simulink model "rlMADDPG4PFC2"  (R2024b)
settings: Solver=FixedStepAuto  StartTime=0.0  StopTime=Tf  FixedStep=0.001  RelTol=1e-3
StartFcn:
  | %scopes= find_system(bdroot,'BlockType','Scope');
  | %for i = 1:length(scopes)
  | %set_param(scopes{i},'Open','on');
  | %end
values from neighbouring files (symbols this model uses):
  amax_ego = 0.4    [MADDPG4_1.m]    (also in MADDPG4__no_rules.m; RL_COMP.m)
  amin_ego = -0.5    [MADDPG4_1.m]    (also in MADDPG4__no_rules.m; RL_COMP.m)
  Cf = 19000    [MADDPG4_1.m]    (also in MADDPG4__no_rules.m; RL_COMP.m)
  Cr = 33000    [MADDPG4_1.m]    (also in MADDPG4__no_rules.m; RL_COMP.m)
  D_default = 1.5    [MADDPG4_1.m]    (also in MADDPG4__no_rules.m; RL_COMP.m)
  e1_initial = 0    [MADDPG4_1.m]    (also in MADDPG4__no_rules.m = -0.05; RL_COMP.m = -0.05)
  e2_initial = 0.26    [MADDPG4_1.m]    (also in MADDPG4__no_rules.m = 0.05; RL_COMP.m = 0.05)
  Iz = 2875    [MADDPG4_1.m]    (also in MADDPG4__no_rules.m; RL_COMP.m)
  lf = 1.4    [MADDPG4_1.m]    (also in MADDPG4__no_rules.m; RL_COMP.m)
  lr = 1.6    [MADDPG4_1.m]    (also in MADDPG4__no_rules.m; RL_COMP.m)
  m = 1600    [MADDPG4_1.m]    (also in MADDPG4__no_rules.m; RL_COMP.m)
  t_gap = 1.4    [MADDPG4_1.m]    (also in MADDPG4__no_rules.m; RL_COMP.m)
  target = 3    [MADDPG4_1.m]    (also in MADDPG4__no_rules.m; RL_COMP.m = 1)
  tau = 0.5    [MADDPG4_1.m]    (also in MADDPG4__no_rules.m; RL_COMP.m)
  Ts = 0.1    [MADDPG4_1.m]    (also in MADDPG4__no_rules.m; RL_COMP.m)
  umax_ego = 0.2618    [MADDPG4_1.m]    (also in MADDPG4__no_rules.m; RL_COMP.m)
  umin_ego = -0.2618    [MADDPG4_1.m]    (also in MADDPG4__no_rules.m; RL_COMP.m)
  v0_FV1 = 0.5    [MADDPG4_1.m]    (also in MADDPG4__no_rules.m; RL_COMP.m)
  v0_FV2 = 0.5    [MADDPG4_1.m]    (also in MADDPG4__no_rules.m; RL_COMP.m)
  v0_LV = 0.9    [MADDPG4_1.m]    (also in MADDPG4__no_rules.m; RL_COMP.m)
  v_set = 1.5    [MADDPG4_1.m]    (also in MADDPG4__no_rules.m; RL_COMP.m)
  x0_FV1 = 1.5    [MADDPG4_1.m]    (also in MADDPG4__no_rules.m; RL_COMP.m)
  x0_FV2 = 0    [MADDPG4_1.m]    (also in MADDPG4__no_rules.m; RL_COMP.m)
  x0_LV = 3    [MADDPG4_1.m]    (also in MADDPG4__no_rules.m; RL_COMP.m)
undefined symbols (not defined in the file or in its folder): DiscIntNeverNeededParam, Speed, SteeringAngle
libraries: simulink x19, rllib x4, robotlib x4, dspfdesign x2
(part 1 of 2)
settings Model: Creator=The MathWorks, Inc.  LastModifiedBy=Leegh
settings SolverCC: AlgebraicLoopSolver=TrustRegion
settings DataIOCC: SaveOutput=off  SignalLogging=off  DSMLogging=off  SaveTime=off  ReturnWorkspaceOutputs=off
settings OptimizationCC: ReuseModelBlockBuffer=off
settings DebuggingCC: ParameterPrecisionLossMsg=none  UnconnectedInputMsg=warning  UnconnectedOutputMsg=warning  UnconnectedLineMsg=warning  ArithmeticOperatorsInVariantConditions=warning
settings ModelReferenceCC: EnableRefExpFcnMdlSchedulingChecks=on
settings SFSimCC: SimUseLocalCustomCode=off
settings RTWCC: RTWUseLocalCustomCode=off  GPUComputeCapability=3.5

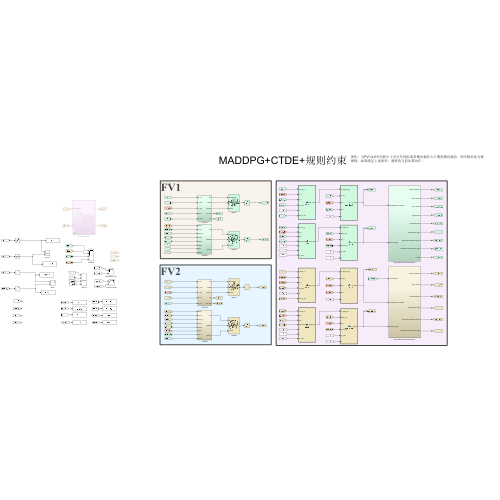
[thumbnail: Simulink's stored preview of the top-level diagram]
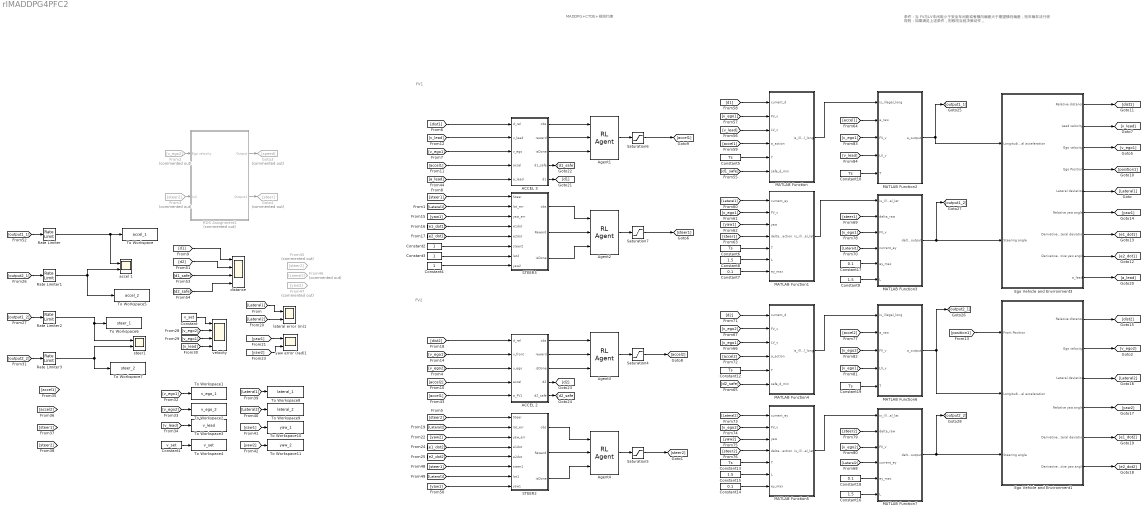
== system rlMADDPG4PFC2 ==
  note: FV2
  note: FV1
  note: MADDPG+CTDE+规则约束
  note: 条件：当 FV与LV车间距小于安全车间距或者横向偏差大于期望横向偏差，则车辆非法行驶
      | 规则：如果满足上述条件，则修改当前决策动作 。
  ACCEL 2 : Subsystem
  ACCEL 3 : Subsystem
  Agent1 : rllib/RL Agent  Agent=agent1  ExternalActionAsInput=off  ProvideLastAction=off  ProvideCumRwd=off  TreatAsDirectFeedthrough=on  UseStrictObservationDataTypes=off
  Agent2 : rllib/RL Agent  Agent=agent2  ExternalActionAsInput=off  ProvideLastAction=off  ProvideCumRwd=off  TreatAsDirectFeedthrough=on  UseStrictObservationDataTypes=off
  Agent3 : rllib/RL Agent  Agent=agent3  ExternalActionAsInput=off  ProvideLastAction=off  ProvideCumRwd=off  TreatAsDirectFeedthrough=on  UseStrictObservationDataTypes=off
  Agent4 : rllib/RL Agent  Agent=agent4  ExternalActionAsInput=off  ProvideLastAction=off  ProvideCumRwd=off  TreatAsDirectFeedthrough=on  UseStrictObservationDataTypes=off
  Constant : Constant  Value=v_set
  Constant1 : Constant  Value=v_set
  Constant{5..6,10,12..13,19} (6 alike) : Constant  Value=Ts
  Constant{7,14,17..18} (4 alike) : Constant  Value=0.1
  Constant{8..9,15..16} (4 alike) : Constant  Value=1.5
  Constant2 : Constant
  Constant3 : Constant
  Constant4 : Constant
  Ego Vehicle and Environment1 : Subsystem
  Ego Vehicle and Environment3 : Subsystem
  From2 : From  Commented=on  GotoTag=v_ego2
  From3 : From  Commented=on  GotoTag=steer2
  From45 : From  Commented=on  GotoTag=steer2
  From46 : From  Commented=on  GotoTag=Lateral2
  From47 : From  Commented=on  GotoTag=yaw2
  Goto3 : Goto  Commented=on  GotoTag=speed
  Goto4 : Goto  Commented=on  GotoTag=steer
  MATLAB Function : MATLAB Function  TreatAsAtomicUnit=on
  MATLAB Function1 : MATLAB Function  TreatAsAtomicUnit=on
  MATLAB Function2 : MATLAB Function  TreatAsAtomicUnit=on
  MATLAB Function3 : MATLAB Function  TreatAsAtomicUnit=on
  MATLAB Function4 : MATLAB Function  TreatAsAtomicUnit=on
  MATLAB Function5 : MATLAB Function  TreatAsAtomicUnit=on
  MATLAB Function6 : MATLAB Function  TreatAsAtomicUnit=on
  MATLAB Function7 : MATLAB Function  TreatAsAtomicUnit=on
  ROS Assignment1 : Subsystem  Commented=on
  Rate Limiter : RateLimiter  RisingSlewLimit=0.8  FallingSlewLimit=-0.8  SampleTimeMode=inherited
  Rate Limiter1 : RateLimiter  RisingSlewLimit=0.8  FallingSlewLimit=-0.8  SampleTimeMode=inherited
  Rate Limiter2 : RateLimiter  RisingSlewLimit=0.25  FallingSlewLimit=-0.25  SampleTimeMode=inherited
  Rate Limiter3 : RateLimiter  RisingSlewLimit=0.25  FallingSlewLimit=-0.25  SampleTimeMode=inherited
  STEER2 : Subsystem
  STEER3 : Subsystem
  Saturation4 : Saturate  UpperLimit=amax_ego  LowerLimit=amin_ego
  Saturation5 : Saturate  UpperLimit=umax_ego  LowerLimit=umin_ego
  Saturation6 : Saturate  UpperLimit=amax_ego  LowerLimit=amin_ego
  Saturation7 : Saturate  UpperLimit=umax_ego  LowerLimit=umin_ego
  To Workspace : ToWorkspace  VariableName=accel_1  SampleTime=-1
      settings: Save2DSignal=2-D array (concatenate along first dimension)
  To Workspace1 : ToWorkspace  VariableName=v_ego_1  SampleTime=-1
      settings: Save2DSignal=2-D array (concatenate along first dimension)
  To Workspace10 : ToWorkspace  VariableName=yaw_1  SampleTime=-1
      settings: Save2DSignal=2-D array (concatenate along first dimension)
  To Workspace11 : ToWorkspace  VariableName=yaw_2  SampleTime=-1
      settings: Save2DSignal=2-D array (concatenate along first dimension)
  To Workspace2 : ToWorkspace  VariableName=v_ego_2  SampleTime=-1
      settings: Save2DSignal=2-D array (concatenate along first dimension)
  To Workspace3 : ToWorkspace  VariableName=v_lead  SampleTime=-1
      settings: Save2DSignal=2-D array (concatenate along first dimension)
  To Workspace4 : ToWorkspace  VariableName=v_set  SampleTime=-1
      settings: Save2DSignal=2-D array (concatenate along first dimension)
  To Workspace5 : ToWorkspace  VariableName=accel_2  SampleTime=-1
      settings: Save2DSignal=2-D array (concatenate along first dimension)
  To Workspace6 : ToWorkspace  VariableName=steer_1  SampleTime=-1
      settings: Save2DSignal=2-D array (concatenate along first dimension)
  To Workspace7 : ToWorkspace  VariableName=steer_2  SampleTime=-1
      settings: Save2DSignal=2-D array (concatenate along first dimension)
  To Workspace8 : ToWorkspace  VariableName=lateral_1  SampleTime=-1
      settings: Save2DSignal=2-D array (concatenate along first dimension)
  To Workspace9 : ToWorkspace  VariableName=lateral_2  SampleTime=-1
      settings: Save2DSignal=2-D array (concatenate along first dimension)
  accel 1 : Scope  NumInputPorts=2
  distance : Scope  NumInputPorts=4
  lateral error (m)1 : Scope  NumInputPorts=2
  steer1 : Scope  NumInputPorts=2
  velocity : Scope  NumInputPorts=4
  yaw error (rad)1 : Scope  NumInputPorts=2
  wires:
  Ego Vehicle and Environment1/2(Ego velocity) -> [v_ego2]
  [Lateral2] -> STEER2/2(lat_err)
  [e1_dot1] -> STEER3/4("e1dot ")
  Ego Vehicle and Environment3/5(Lateral deviation) -> [Lateral1]
  Agent3/1 -> Saturation4/1
  ACCEL 3/2(reward) -> Agent1/2
  From2/1 -> ROS Assignment1/1(Ego velocity)
  Ego Vehicle and Environment3/2(Lead velocity) -> [v_lead]
  [steer1] -> STEER3/1(Steer)
  Ego Vehicle and Environment3/1(Relative distance) -> [dist1]
  Ego Vehicle and Environment1/5(Derivative of lateral deviation) -> [e1_dot2]
  [dist1] -> ACCEL 3/1(d_rel)
  Ego Vehicle and Environment1/4(Relative yaw angle) -> [yaw2]
  [yaw2] -> STEER2/3(yaw_err)
  Saturation4/1 -> [accel2]
  [dist2] -> ACCEL 2/1(d_rel)
  Ego Vehicle and Environment3/6(Relative yaw angle) -> [yaw1]
  Ego Vehicle and Environment3/7(Derivative of lateral deviation) -> [e1_dot1]
  ROS Assignment1/2(Output1) -> Goto4/1
  [position1] -> Ego Vehicle and Environment1/1(Front Position)
  Agent1/1 -> Saturation6/1
  [accel1] -> ACCEL 3/4(accel)
  [e2_dot1] -> STEER3/5(e2dot)
  [v_lead] -> ACCEL 3/2(v_lead)
  Ego Vehicle and Environment3/3(Ego velocity) -> [v_ego1]
  STEER3/3(isDone) -> Agent2/3
  Ego Vehicle and Environment3/8(Derivative of relative yaw angle) -> [e2_dot1]
  STEER3/1(obs) -> Agent2/1
  [v_ego2] -> ACCEL 2/3(v_ego)
  [yaw1] -> STEER3/3(yaw_err)
  [v_ego1] -> ACCEL 3/3(v_ego)
  Ego Vehicle and Environment1/6(Derivative of relative yaw angle) -> [e2_dot2]
  [v_ego1] -> ACCEL 2/2(v_front)
  STEER3/2(Reward) -> Agent2/2
  [steer2] -> STEER2/1(Steer)
  From3/1 -> ROS Assignment1/2(In2)
  ACCEL 2/1(obs) -> Agent3/1
  Agent2/1 -> Saturation7/1
  Ego Vehicle and Environment3/4(Ego Position) -> [position1]
  Saturation6/1 -> [accel1]
  ACCEL 2/3(isDone) -> Agent3/3
  STEER2/2(Reward) -> Agent4/2
  [Lateral1] -> STEER3/2(lat_err)
  ACCEL 3/1(obs) -> Agent1/1
  STEER2/1(obs) -> Agent4/1
  ACCEL 3/3(isDone) -> Agent1/3
  ROS Assignment1/1(Output) -> Goto3/1
  Ego Vehicle and Environment1/1(Relative distance) -> [dist2]
  [e2_dot2] -> STEER2/5(e2dot)
  Saturation5/1 -> [steer2]
  STEER2/3(isDone) -> Agent4/3
  Agent4/1 -> Saturation5/1
  Ego Vehicle and Environment1/3(Lateral deviation) -> [Lateral2]
  Saturation7/1 -> [steer1]
  [accel2] -> ACCEL 2/4(accel)
  [e1_dot2] -> STEER2/4("e1dot ")
  ACCEL 2/2(reward) -> Agent3/2
  Ego Vehicle and Environment3/9(a_lead) -> [a_lead]
  [a_lead] -> ACCEL 3/5(a_lead)
  [accel1] -> ACCEL 2/5(a_FV1)
  Constant2/1 -> STEER3/6(steer2)
  Constant3/1 -> STEER3/7(lat2)
  Constant4/1 -> STEER3/8(yaw2)
  [steer1] -> STEER2/6(steer1)
  [Lateral1] -> STEER2/7(lat1)
  [yaw1] -> STEER2/8(yaw1)
  [Lateral1] -> lateral error (m)1/1
  [v_ego2] -> To Workspace2/1
  [yaw2] -> yaw error (rad)1/2
  [v_ego1] -> velocity/3
  [output1_2] -> Rate Limiter2/1
  [output2_1] -> Rate Limiter1/1
  [v_lead] -> velocity/4
  [v_lead] -> To Workspace3/1
  Constant/1 -> velocity/1
  [Lateral2] -> lateral error (m)1/2
  [output1_1] -> Rate Limiter/1
  [d1] -> distance/1
  [d2] -> distance/2
  [yaw2] -> To Workspace11/1
  [v_ego1] -> To Workspace1/1
  [v_ego2] -> velocity/2
  [yaw1] -> yaw error (rad)1/1
  Constant1/1 -> To Workspace4/1
  [yaw1] -> To Workspace10/1
  [Lateral2] -> To Workspace9/1
  [output2_2] -> Rate Limiter3/1
  [Lateral1] -> To Workspace8/1
  ACCEL 3/5(d1) -> [d1]
  ACCEL 3/4(d1_safe) -> [d1_safe]
  ACCEL 2/4(d2) -> [d2]
  ACCEL 2/5(d2_safe) -> [d2_safe]
  [d1_safe] -> distance/3
  [d2_safe] -> distance/4
  Constant5/1 -> MATLAB Function/5(T)
  [d1_safe] -> MATLAB Function/6(safe_d_min)
  [v_lead] -> MATLAB Function/3(LV_v)
  [v_ego1] -> MATLAB Function/2(FV_v)
  [d1] -> MATLAB Function/1(current_d)
  [accel1] -> MATLAB Function/4(a_action)
  [Lateral1] -> MATLAB Function1/1(current_ey)
  [v_ego1] -> MATLAB Function1/2(FV_v)
  [yaw1] -> MATLAB Function1/3(yaw)
  [steer1] -> MATLAB Function1/4(delta_action)
  Constant6/1 -> MATLAB Function1/5(T)
  Constant8/1 -> MATLAB Function1/6(L)
  Constant7/1 -> MATLAB Function1/7(ey_max)
  MATLAB Function2/1(a_output) -> [output1_1], Ego Vehicle and Environment3/1(Longitudinal acceleration)
  MATLAB Function3/1(delta_output) -> [output1_2], Ego Vehicle and Environment3/2(Steering angle)
  MATLAB Function6/1(a_output) -> [output2_1], Ego Vehicle and Environment1/2(Longitudinal acceleration)
  MATLAB Function7/1(delta_output) -> [output2_2], Ego Vehicle and Environment1/3(Steering angle)
  MATLAB Function/1(is_illegal_long) -> MATLAB Function2/1(is_illegal_long)
  [accel1] -> MATLAB Function2/2(a_raw)
  MATLAB Function1/1(is_illegal_lat) -> MATLAB Function3/1(is_illegal_lat)
  [steer1] -> MATLAB Function3/2(delta_raw)
  [steer2] -> MATLAB Function7/2(delta_raw)
  MATLAB Function5/1(is_illegal_lat) -> MATLAB Function7/1(is_illegal_lat)
  MATLAB Function4/1(is_illegal_long) -> MATLAB Function6/1(is_illegal_long)
  Constant14/1 -> MATLAB Function5/7(ey_max)
  Constant15/1 -> MATLAB Function5/6(L)
  Constant13/1 -> MATLAB Function5/5(T)
  [steer2] -> MATLAB Function5/4(delta_action)
  [yaw2] -> MATLAB Function5/3(yaw)
  [v_ego2] -> MATLAB Function5/2(FV_v)
  [Lateral2] -> MATLAB Function5/1(current_ey)
  [accel2] -> MATLAB Function4/4(a_action)
  [d2] -> MATLAB Function4/1(current_d)
  [v_ego2] -> MATLAB Function4/2(FV_v)
  [v_ego1] -> MATLAB Function4/3(LV_v)
  [d2_safe] -> MATLAB Function4/6(safe_d_min)
  Constant12/1 -> MATLAB Function4/5(T)
  [accel2] -> MATLAB Function6/2(a_raw)
  Constant9/1 -> MATLAB Function3/6(L)
  Constant17/1 -> MATLAB Function3/5(ey_max)
  Constant18/1 -> MATLAB Function7/5(ey_max)
  [Lateral2] -> MATLAB Function7/4(current_ey)
  [Lateral1] -> MATLAB Function3/4(current_ey)
  [v_ego1] -> MATLAB Function3/3(FV_v)
  [v_ego2] -> MATLAB Function7/3(FV_v)
  Constant16/1 -> MATLAB Function7/6(L)
  Constant19/1 -> MATLAB Function6/5(T)
  [v_ego1] -> MATLAB Function6/4(LV_v)
  [v_ego2] -> MATLAB Function6/3(FV_v)
  Constant10/1 -> MATLAB Function2/5(T)
  [v_ego1] -> MATLAB Function2/3(FV_v)
  [v_lead] -> MATLAB Function2/4(LV_v)
  Rate Limiter/1 -> To Workspace/1, accel 1/1
  Rate Limiter1/1 -> accel 1/2, To Workspace5/1
  Rate Limiter2/1 -> To Workspace6/1, steer1/1
  Rate Limiter3/1 -> steer1/2, To Workspace7/1

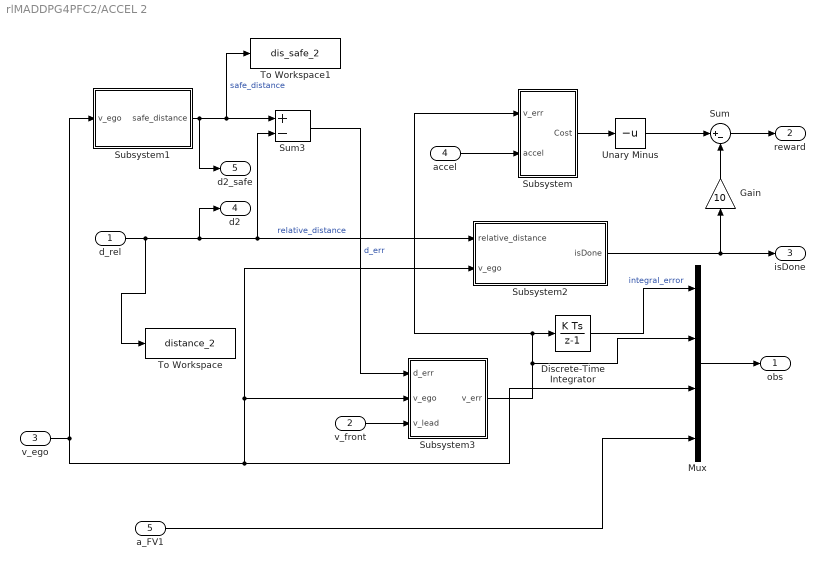
== system rlMADDPG4PFC2/ACCEL 2 ==
  d_rel : Inport
  v_front : Inport  Port=2
  v_ego : Inport  Port=3
  accel : Inport  Port=4
  a_FV1 : Inport  Port=5
  Discrete-Time Integrator : DiscreteIntegrator  SampleTime=-1  ICPrevOutput=DiscIntNeverNeededParam  ICPrevScaledInput=DiscIntNeverNeededParam
  Gain : Gain  Gain=10
  Mux : Mux
  Subsystem : Subsystem
  Subsystem1 : Subsystem
  Subsystem2 : Subsystem
  Subsystem3 : Subsystem
  Sum : Sum  Inputs=|+-
  Sum3 : Sum  Inputs=+-
  To Workspace : ToWorkspace  VariableName=distance_2  SampleTime=-1
      settings: Save2DSignal=2-D array (concatenate along first dimension)
  To Workspace1 : ToWorkspace  VariableName=dis_safe_2  SampleTime=-1
      settings: Save2DSignal=2-D array (concatenate along first dimension)
  Unary Minus : UnaryMinus
  obs : Outport  VectorParamsAs1DForOutWhenUnconnected=off
  reward : Outport  Port=2  VectorParamsAs1DForOutWhenUnconnected=off
  isDone : Outport  Port=3  VectorParamsAs1DForOutWhenUnconnected=off
  d2 : Outport  Port=4  VectorParamsAs1DForOutWhenUnconnected=off
  d2_safe : Outport  Port=5  VectorParamsAs1DForOutWhenUnconnected=off
  wires:
  v_front/1 -> Subsystem3/3(v_lead)
  Discrete-Time Integrator/1 -> Mux/1  "integral_error"
  Mux/1 -> obs/1
  v_ego/1 -> Subsystem3/2(v_ego), Subsystem2/2(v_ego), Mux/3, Subsystem1/1(v_ego)
  d_rel/1 -> To Workspace/1, d2/1, Sum3/2, Subsystem2/1(relative_distance)  "relative_distance"
  Subsystem/1(Cost) -> Unary Minus/1
  Sum3/1 -> Subsystem3/1(d_err)  "d_err"
  Subsystem1/1(safe_distance) -> d2_safe/1, To Workspace1/1, Sum3/1  "safe_distance"
  accel/1 -> Subsystem/2(accel)
  Subsystem3/1(v_err) -> Mux/2, Subsystem/1(v_err), Discrete-Time Integrator/1
  Subsystem2/1(isDone) -> isDone/1, Gain/1
  Unary Minus/1 -> Sum/1
  Gain/1 -> Sum/2
  Sum/1 -> reward/1
  a_FV1/1 -> Mux/4

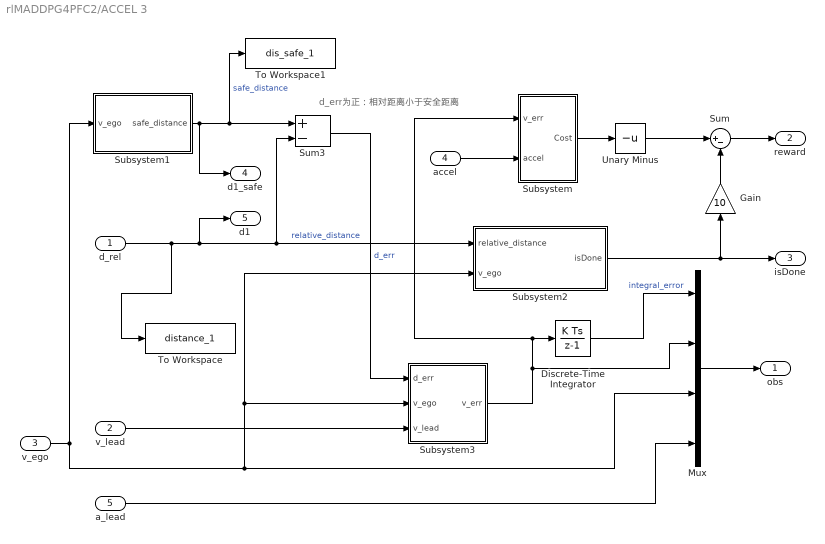
== system rlMADDPG4PFC2/ACCEL 3 ==
  note: d_err为正：相对距离小于安全距离
  d_rel : Inport
  v_lead : Inport  Port=2
  v_ego : Inport  Port=3
  accel : Inport  Port=4
  a_lead : Inport  Port=5
  Discrete-Time Integrator : DiscreteIntegrator  SampleTime=-1  ICPrevOutput=DiscIntNeverNeededParam  ICPrevScaledInput=DiscIntNeverNeededParam
  Gain : Gain  Gain=10
  Mux : Mux
  Subsystem : Subsystem
  Subsystem1 : Subsystem
  Subsystem2 : Subsystem
  Subsystem3 : Subsystem
  Sum : Sum  Inputs=|+-
  Sum3 : Sum  Inputs=+-
  To Workspace : ToWorkspace  VariableName=distance_1  SampleTime=-1
      settings: Save2DSignal=2-D array (concatenate along first dimension)
  To Workspace1 : ToWorkspace  VariableName=dis_safe_1  SampleTime=-1
      settings: Save2DSignal=2-D array (concatenate along first dimension)
  Unary Minus : UnaryMinus
  obs : Outport  VectorParamsAs1DForOutWhenUnconnected=off
  reward : Outport  Port=2  VectorParamsAs1DForOutWhenUnconnected=off
  isDone : Outport  Port=3  VectorParamsAs1DForOutWhenUnconnected=off
  d1_safe : Outport  Port=4  VectorParamsAs1DForOutWhenUnconnected=off
  d1 : Outport  Port=5  VectorParamsAs1DForOutWhenUnconnected=off
  wires:
  v_lead/1 -> Subsystem3/3(v_lead)
  Discrete-Time Integrator/1 -> Mux/1  "integral_error"
  Mux/1 -> obs/1
  v_ego/1 -> Subsystem3/2(v_ego), Subsystem2/2(v_ego), Mux/3, Subsystem1/1(v_ego)
  d_rel/1 -> To Workspace/1, d1/1, Sum3/2, Subsystem2/1(relative_distance)  "relative_distance"
  Subsystem/1(Cost) -> Unary Minus/1
  Sum3/1 -> Subsystem3/1(d_err)  "d_err"
  Subsystem1/1(safe_distance) -> d1_safe/1, To Workspace1/1, Sum3/1  "safe_distance"
  accel/1 -> Subsystem/2(accel)
  Subsystem3/1(v_err) -> Mux/2, Subsystem/1(v_err), Discrete-Time Integrator/1
  Subsystem2/1(isDone) -> isDone/1, Gain/1
  Unary Minus/1 -> Sum/1
  Gain/1 -> Sum/2
  Sum/1 -> reward/1
  a_lead/1 -> Mux/4

== system rlMADDPG4PFC2/Ego Vehicle and Environment1 ==
  Front Position : Inport
  Longitudinal acceleration : Inport  Port=2
  Steering angle : Inport  Port=3
  Ego sensor : Subsystem
  Ego vehicle : Subsystem
  Initial ego position : Constant  Value=x0_FV2
  Initial lateral deviation : Constant  Value=e1_initial
  Initial relative yaw angle : Constant  Value=e2_initial
  Sum3 : Sum  Inputs=+-
  curvature1 : Subsystem
  Relative distance : Outport  VectorParamsAs1DForOutWhenUnconnected=off
  Ego velocity : Outport  Port=2  VectorParamsAs1DForOutWhenUnconnected=off
  Lateral deviation : Outport  Port=3  VectorParamsAs1DForOutWhenUnconnected=off
  Relative yaw angle : Outport  Port=4  VectorParamsAs1DForOutWhenUnconnected=off
  Derivative of lateral deviation : Outport  Port=5  VectorParamsAs1DForOutWhenUnconnected=off
  Derivative of relative yaw angle : Outport  Port=6  VectorParamsAs1DForOutWhenUnconnected=off
  wires:
  Front Position/1 -> Sum3/1
  Longitudinal acceleration/1 -> Ego vehicle/1(Acceleration)  "acceleration"
  Initial ego position/1 -> Ego vehicle/3(Initial position)
  Ego sensor/4(e2_dot) -> Derivative of relative yaw angle/1
  Ego sensor/3(e1_dot) -> Derivative of lateral deviation/1
  Sum3/1 -> Relative distance/1
  curvature1/1(curvature) -> Ego sensor/4(Curvature)
  Initial relative yaw angle/1 -> Ego sensor/5(Initial relative yaw angle)
  Ego sensor/2(Relative yaw angle) -> Relative yaw angle/1
  Ego vehicle/4(Yaw Rate) -> Ego sensor/3(Yaw rate)
  Ego vehicle/1(Position) -> curvature1/1(position), Sum3/2
  Ego sensor/1(Lateral deviation) -> Lateral deviation/1
  Steering angle/1 -> Ego vehicle/2(Steering)  "steering"
  Ego vehicle/2(Longitudinal Velocity) -> Ego velocity/1, Ego sensor/1(Longitudinal velocity)
  Initial lateral deviation/1 -> Ego sensor/6(Initial lateral deviation)
  Ego vehicle/3(Lateral Velocity) -> Ego sensor/2(Lateral velocity)

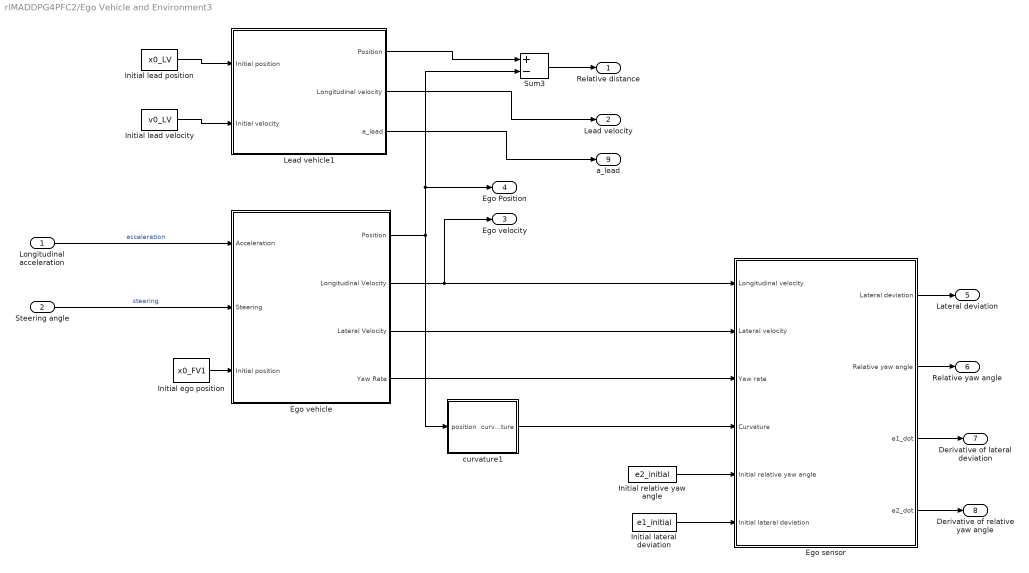
== system rlMADDPG4PFC2/Ego Vehicle and Environment3 ==
  Longitudinal acceleration : Inport
  Steering angle : Inport  Port=2
  Ego sensor : Subsystem
  Ego vehicle : Subsystem
  Initial ego position : Constant  Value=x0_FV1
  Initial lateral deviation : Constant  Value=e1_initial
  Initial lead position : Constant  Value=x0_LV
  Initial lead velocity : Constant  Value=v0_LV
  Initial relative yaw angle : Constant  Value=e2_initial
  Lead vehicle1 : Subsystem
  Sum3 : Sum  Inputs=+-
  curvature1 : Subsystem
  Relative distance : Outport  VectorParamsAs1DForOutWhenUnconnected=off
  Lead velocity : Outport  Port=2  VectorParamsAs1DForOutWhenUnconnected=off
  Ego velocity : Outport  Port=3  VectorParamsAs1DForOutWhenUnconnected=off
  Ego Position : Outport  Port=4
  Lateral deviation : Outport  Port=5  VectorParamsAs1DForOutWhenUnconnected=off
  Relative yaw angle : Outport  Port=6  VectorParamsAs1DForOutWhenUnconnected=off
  Derivative of lateral deviation : Outport  Port=7  VectorParamsAs1DForOutWhenUnconnected=off
  Derivative of relative yaw angle : Outport  Port=8  VectorParamsAs1DForOutWhenUnconnected=off
  a_lead : Outport  Port=9  VectorParamsAs1DForOutWhenUnconnected=off
  wires:
  Lead vehicle1/1(Position) -> Sum3/1
  Ego sensor/4(e2_dot) -> Derivative of relative yaw angle/1
  Initial lead velocity/1 -> Lead vehicle1/2(Initial velocity)
  Ego vehicle/3(Lateral Velocity) -> Ego sensor/2(Lateral velocity)
  Sum3/1 -> Relative distance/1
  Initial lead position/1 -> Lead vehicle1/1(Initial position)
  Ego vehicle/1(Position) -> curvature1/1(position), Ego Position/1, Sum3/2
  Ego sensor/3(e1_dot) -> Derivative of lateral deviation/1
  Lead vehicle1/2(Longitudinal velocity) -> Lead velocity/1
  Ego sensor/1(Lateral deviation) -> Lateral deviation/1
  Steering angle/1 -> Ego vehicle/2(Steering)  "steering"
  Initial lateral deviation/1 -> Ego sensor/6(Initial lateral deviation)
  Ego sensor/2(Relative yaw angle) -> Relative yaw angle/1
  Ego vehicle/2(Longitudinal Velocity) -> Ego velocity/1, Ego sensor/1(Longitudinal velocity)
  Initial ego position/1 -> Ego vehicle/3(Initial position)
  curvature1/1(curvature) -> Ego sensor/4(Curvature)
  Ego vehicle/4(Yaw Rate) -> Ego sensor/3(Yaw rate)
  Initial relative yaw angle/1 -> Ego sensor/5(Initial relative yaw angle)
  Longitudinal acceleration/1 -> Ego vehicle/1(Acceleration)  "acceleration"
  Lead vehicle1/3(a_lead) -> a_lead/1

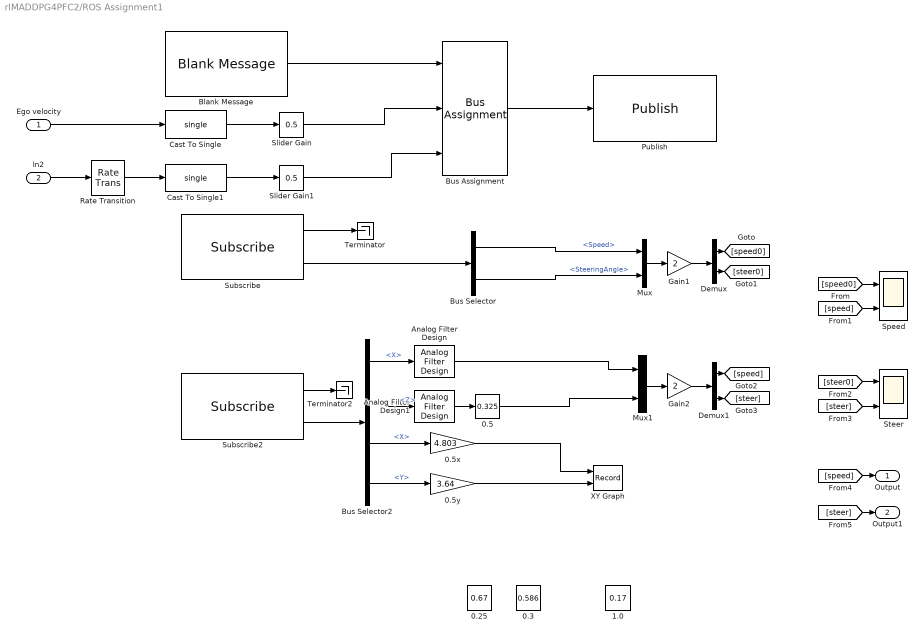
== system rlMADDPG4PFC2/ROS Assignment1 ==
  Ego velocity : Inport
  In2 : Inport  Port=2
  0.25 : simulink/Math Operations/Slider Gain  gain=0.67  low=0  high=2
  0.3 : simulink/Math Operations/Slider Gain  gain=0.586  low=0  high=2
  0.5 : simulink/Math Operations/Slider Gain  gain=0.325  low=0  high=2
  0.5x : Gain  Gain=4.803
  0.5y : Gain  Gain=3.64
  1.0 : simulink/Math Operations/Slider Gain  gain=0.17  low=0  high=2
  Analog Filter Design : dspfdesign/Analog Filter Design  method=Butterworth  filttype=Lowpass  N=8  Wlo=30  Whi=80  Rp=2  Rs=40
  Analog Filter Design1 : dspfdesign/Analog Filter Design  method=Butterworth  filttype=Lowpass  N=8  Wlo=50  Whi=80  Rp=2  Rs=40
  Blank Message : robotlib/Blank Message  messageClass=Message  entityType=ackermann_msgs/AckermannDrive  messageType=ackermann_msgs/AckermannDrive  SampleTime=inf  legacyBusStruct=off
  Bus Assignment : BusAssignment  AssignedSignals=Speed,SteeringAngle
  Bus Selector : BusSelector  OutputSignals=Speed,SteeringAngle
  Bus Selector2 : BusSelector  OutputSignals=Twist.Twist.Linear.X,Twist.Twist.Angular.Z,Pose.Pose.Position.X,Pose.Pose.Position.Y
  Cast To Single : DataTypeConversion  OutDataTypeStr=single  SaturateOnIntegerOverflow=off  RndMeth=Floor
  Cast To Single1 : DataTypeConversion  OutDataTypeStr=single  SaturateOnIntegerOverflow=off  RndMeth=Floor
  Demux : Demux  Outputs=2
  Demux1 : Demux  Outputs=2
  Gain1 : Gain  Gain=2
  Gain2 : Gain  Gain=2
  Mux : Mux  Inputs=2
  Mux1 : Mux  Inputs=2
  Publish : robotlib/Publish  topicSource=Select from ROS network  topic=/tianracer/ackermann_cmd  messageType=ackermann_msgs/AckermannDrive  legacyBusStruct=off  messageQueueLength=1
  Rate Transition : RateTransition
  Slider Gain : simulink/Math Operations/Slider Gain  gain=0.5  low=0  high=2
  Slider Gain1 : simulink/Math Operations/Slider Gain  gain=0.5  low=0  high=2
  Speed : Scope  NumInputPorts=2
  Steer : Scope  NumInputPorts=2
  Subscribe : robotlib/Subscribe  topicSource=Select from ROS network  topic=/tianracer/ackermann_cmd  messageType=ackermann_msgs/AckermannDrive  SampleTime=-1  legacyBusStruct=off  messageQueueLength=1
  Subscribe2 : robotlib/Subscribe  topicSource=Select from ROS network  topic=/tianracer/odom  messageType=nav_msgs/Odometry  SampleTime=-1  legacyBusStruct=off  messageQueueLength=1
  Terminator : Terminator
  Terminator2 : Terminator
  XY Graph : Record  FileSettingsInternal="{\"entries\":[{\"content\":{\"excelSettings\":{\"content\":{},\"type\":\"Streamout.ExcelSettings\"}},\"type\":\"Streamout.FileSettingStorage\",\"uuid\":\"\"}],\"packageUris\":[\"http:\\/\\/schema.mathworks.com\\/mf0\\/streamout_blocks\\/R2020a\"],\"version\":\"1.0\"}"  Layout=[1 1]  SignalsInternal="{\"entries\":[{\"content\":{\"signals\":[{\"content\":{\"blockPath\":[],\"dimensions\":[1],\"domain\":\"\",\"lineColor\":\"#77ac30\",\"plots\":[ 1 ],\"port\":1,\"signalID\":1,\"signalName\":\"0.5x\"},\"type\":\"RecordBlkView.Signal\",\"uuid\":\"\"},{\"content\":{\"blockPath\":[],\"dimensions\":[1],\"domain\":\"\",\"lineColor\":\"#ff6929\",\"plots\":[ 1 ],\"port\":2,\"signalID\":2,\"signalName\":\"0.5y\"},\"type\":\"RecordBlkView.Signal\",\"uuid\":\"\"}]},\"type\":\"RecordBlkView.InputSignals\",\"uuid\":\"\"}],\"packageUris\":[\"http:\\/\\/schema.mathworks.com\\/mf0\\/streamout_blocks\\/R2020a\"],\"version\":\"1.0\"}"  CompatibilityTag=XY
  Output : Outport
  Output1 : Outport  Port=2
  wires:
  Subscribe/1 -> Terminator/1
  Slider Gain/1 -> Bus Assignment/2
  Subscribe/2 -> Bus Selector/1
  Bus Selector/2 -> Mux/2  "<SteeringAngle>"
  Cast To Single/1 -> Slider Gain/1
  Cast To Single1/1 -> Slider Gain1/1
  Slider Gain1/1 -> Bus Assignment/3
  Bus Selector/1 -> Mux/1  "<Speed>"
  Bus Assignment/1 -> Publish/1
  Blank Message/1 -> Bus Assignment/1
  In2/1 -> Rate Transition/1
  Rate Transition/1 -> Cast To Single1/1
  Ego velocity/1 -> Cast To Single/1
  Subscribe2/2 -> Bus Selector2/1
  Subscribe2/1 -> Terminator2/1
  Bus Selector2/1 -> Analog Filter Design/1  "<X>"
  Bus Selector2/2 -> Analog Filter Design1/1  "<Z>"
  Analog Filter Design1/1 -> 0.5/1
  Bus Selector2/3 -> 0.5x/1  "<X>"
  Bus Selector2/4 -> 0.5y/1  "<Y>"
  Analog Filter Design/1 -> Mux1/1
  0.5/1 -> Mux1/2
  Mux/1 -> Gain1/1
  Gain1/1 -> Demux/1
  Gain2/1 -> Demux1/1
  Mux1/1 -> Gain2/1
  Demux/1 -> [speed0]
  Demux/2 -> [steer0]
  Demux1/1 -> [speed]
  Demux1/2 -> [steer]
  [speed0] -> Speed/1
  [speed] -> Speed/2
  [steer0] -> Steer/1
  [steer] -> Steer/2
  [speed] -> Output/1
  [steer] -> Output1/1
  0.5x/1 -> XY Graph/1
  0.5y/1 -> XY Graph/2

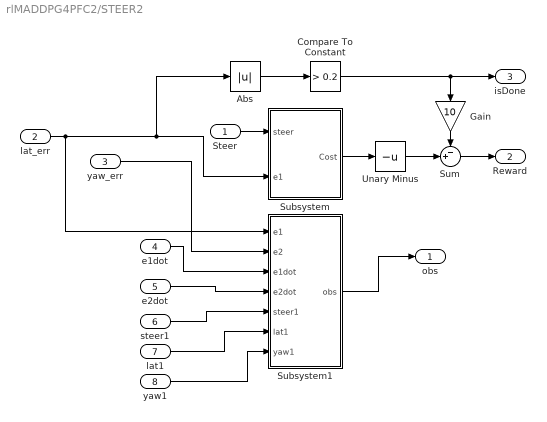
== system rlMADDPG4PFC2/STEER2 ==
  Steer : Inport
  lat_err : Inport  Port=2
  yaw_err : Inport  Port=3
  "e1dot " : Inport  Port=4
  e2dot : Inport  Port=5
  steer1 : Inport  Port=6
  lat1 : Inport  Port=7
  yaw1 : Inport  Port=8
  Abs : Abs  SaturateOnIntegerOverflow=off
  Compare To Constant : simulink/Logic and Bit Operations/Compare To Constant  relop=>  const=0.2  OutDataTypeStr=boolean
  Gain : Gain  Gain=10
  Subsystem : Subsystem
  Subsystem1 : Subsystem
  Sum : Sum  Inputs=-+|
  Unary Minus : UnaryMinus
  obs : Outport  VectorParamsAs1DForOutWhenUnconnected=off
  Reward : Outport  Port=2  VectorParamsAs1DForOutWhenUnconnected=off
  isDone : Outport  Port=3  VectorParamsAs1DForOutWhenUnconnected=off
  wires:
  Subsystem/1(Cost) -> Unary Minus/1
  lat_err/1 -> Subsystem1/1(e1), Subsystem/2(e1), Abs/1
  yaw_err/1 -> Subsystem1/2(e2)
  Abs/1 -> Compare To Constant/1
  Subsystem1/1(obs) -> obs/1
  "e1dot "/1 -> Subsystem1/3(e1dot)
  e2dot/1 -> Subsystem1/4(e2dot)
  Steer/1 -> Subsystem/1(steer)
  Compare To Constant/1 -> isDone/1, Gain/1
  Gain/1 -> Sum/1
  Sum/1 -> Reward/1
  Unary Minus/1 -> Sum/2
  steer1/1 -> Subsystem1/5(steer1)
  lat1/1 -> Subsystem1/6(lat1)
  yaw1/1 -> Subsystem1/7(yaw1)

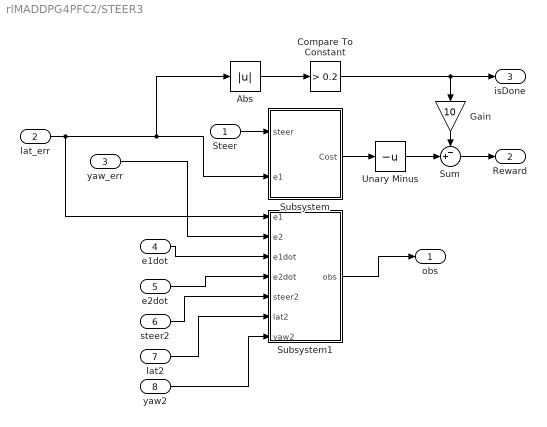
== system rlMADDPG4PFC2/STEER3 ==
  Steer : Inport
  lat_err : Inport  Port=2
  yaw_err : Inport  Port=3
  "e1dot " : Inport  Port=4
  e2dot : Inport  Port=5
  steer2 : Inport  Port=6
  lat2 : Inport  Port=7
  yaw2 : Inport  Port=8
  Abs : Abs  SaturateOnIntegerOverflow=off
  Compare To Constant : simulink/Logic and Bit Operations/Compare To Constant  relop=>  const=0.2  OutDataTypeStr=boolean
  Gain : Gain  Gain=10
  Subsystem : Subsystem
  Subsystem1 : Subsystem
  Sum : Sum  Inputs=-+|
  Unary Minus : UnaryMinus
  obs : Outport  VectorParamsAs1DForOutWhenUnconnected=off
  Reward : Outport  Port=2  VectorParamsAs1DForOutWhenUnconnected=off
  isDone : Outport  Port=3  VectorParamsAs1DForOutWhenUnconnected=off
  wires:
  Subsystem/1(Cost) -> Unary Minus/1
  lat_err/1 -> Subsystem1/1(e1), Subsystem/2(e1), Abs/1
  yaw_err/1 -> Subsystem1/2(e2)
  Abs/1 -> Compare To Constant/1
  Subsystem1/1(obs) -> obs/1
  "e1dot "/1 -> Subsystem1/3(e1dot)
  e2dot/1 -> Subsystem1/4(e2dot)
  Steer/1 -> Subsystem/1(steer)
  Compare To Constant/1 -> isDone/1, Gain/1
  Gain/1 -> Sum/1
  Sum/1 -> Reward/1
  Unary Minus/1 -> Sum/2
  steer2/1 -> Subsystem1/5(steer2)
  lat2/1 -> Subsystem1/6(lat2)
  yaw2/1 -> Subsystem1/7(yaw2)

== system rlMADDPG4PFC2/ACCEL 2/Subsystem ==
  v_err : Inport
  accel : Inport  Port=2
  Compare To Constant : simulink/Logic and Bit Operations/Compare To Constant  relop=<  const=0.09  OutDataTypeStr=boolean
  Gain1 : Gain  Gain=0.1
  Gain2 : Gain  Gain=0.01
  Gain3 : Gain
  Math Function2 : Math  Operator=square  SignedPower=on
  Square : Math  Operator=square  SignedPower=on
  Sum : Sum  Inputs=++-
  Unit Delay : UnitDelay  SampleTime=-1  HasFrameUpgradeWarning=on
  Cost : Outport  VectorParamsAs1DForOutWhenUnconnected=off
  wires:
  v_err/1 -> Square/1
  Math Function2/1 -> Gain1/1
  accel/1 -> Unit Delay/1
  Sum/1 -> Cost/1
  Square/1 -> Compare To Constant/1, Gain2/1
  Unit Delay/1 -> Math Function2/1
  Gain2/1 -> Sum/1
  Gain1/1 -> Sum/2
  Compare To Constant/1 -> Gain3/1
  Gain3/1 -> Sum/3

== system rlMADDPG4PFC2/ACCEL 2/Subsystem1 ==
  v_ego : Inport
  Default Spacing : Constant  Value=D_default  SampleTime=Ts
  Product : Product
  Sum2 : Sum
  Time Gap : Constant  Value=t_gap  SampleTime=Ts
  safe_distance : Outport  VectorParamsAs1DForOutWhenUnconnected=off
  wires:
  Sum2/1 -> safe_distance/1
  Product/1 -> Sum2/2
  Time Gap/1 -> Product/2
  Default Spacing/1 -> Sum2/1
  v_ego/1 -> Product/1

== system rlMADDPG4PFC2/ACCEL 2/Subsystem2 ==
  relative_distance : Inport
  v_ego : Inport  Port=2
  Logical Operator : Logic  Operator=OR  AllPortsSameDT=off  OutDataTypeStr=boolean
  Relative Distance : simulink/Logic and Bit Operations/Compare To Constant  relop=<  const=0  OutDataTypeStr=boolean
  Velocity : simulink/Logic and Bit Operations/Compare To Constant  relop=<  const=0.09  OutDataTypeStr=boolean
  isDone : Outport  VectorParamsAs1DForOutWhenUnconnected=off
  wires:
  Velocity/1 -> Logical Operator/2
  Relative Distance/1 -> Logical Operator/1
  relative_distance/1 -> Relative Distance/1
  Logical Operator/1 -> isDone/1
  v_ego/1 -> Velocity/1

== system rlMADDPG4PFC2/ACCEL 2/Subsystem3 ==
  d_err : Inport
  v_ego : Inport  Port=2
  v_lead : Inport  Port=3
  Constant : Constant  Value=v_set
  Min : MinMax  Inputs=2
  Sum1 : Sum  Inputs=+-
  Switch : Switch  Criteria=u2 > Threshold  SaturateOnIntegerOverflow=off  InputSameDT=off
  v_err : Outport  VectorParamsAs1DForOutWhenUnconnected=off
  wires:
  Sum1/1 -> v_err/1
  v_ego/1 -> Sum1/2
  Switch/1 -> Sum1/1  "v_ref"
  d_err/1 -> Switch/2
  Constant/1 -> Min/2, Switch/3
  Min/1 -> Switch/1
  v_lead/1 -> Min/1

== system rlMADDPG4PFC2/ACCEL 3/Subsystem ==
  v_err : Inport
  accel : Inport  Port=2
  Compare To Constant : simulink/Logic and Bit Operations/Compare To Constant  relop=<  const=0.09  OutDataTypeStr=boolean
  Gain1 : Gain  Gain=0.1
  Gain2 : Gain  Gain=0.01
  Gain3 : Gain
  Math Function2 : Math  Operator=square  SignedPower=on
  Square : Math  Operator=square  SignedPower=on
  Sum : Sum  Inputs=++-
  Unit Delay : UnitDelay  SampleTime=-1  HasFrameUpgradeWarning=on
  Cost : Outport  VectorParamsAs1DForOutWhenUnconnected=off
  wires:
  v_err/1 -> Square/1
  Math Function2/1 -> Gain1/1
  accel/1 -> Unit Delay/1
  Sum/1 -> Cost/1
  Square/1 -> Compare To Constant/1, Gain2/1
  Unit Delay/1 -> Math Function2/1
  Gain2/1 -> Sum/1
  Gain1/1 -> Sum/2
  Compare To Constant/1 -> Gain3/1
  Gain3/1 -> Sum/3

== system rlMADDPG4PFC2/ACCEL 3/Subsystem1 ==
  v_ego : Inport
  Default Spacing : Constant  Value=D_default  SampleTime=Ts
  Product : Product
  Sum2 : Sum
  Time Gap : Constant  Value=t_gap  SampleTime=Ts
  safe_distance : Outport  VectorParamsAs1DForOutWhenUnconnected=off
  wires:
  Sum2/1 -> safe_distance/1
  Product/1 -> Sum2/2
  Time Gap/1 -> Product/2
  Default Spacing/1 -> Sum2/1
  v_ego/1 -> Product/1

== system rlMADDPG4PFC2/ACCEL 3/Subsystem2 ==
  relative_distance : Inport
  v_ego : Inport  Port=2
  Logical Operator : Logic  Operator=OR  AllPortsSameDT=off  OutDataTypeStr=boolean
  Relative Distance : simulink/Logic and Bit Operations/Compare To Constant  relop=<  const=0  OutDataTypeStr=boolean
  Velocity : simulink/Logic and Bit Operations/Compare To Constant  relop=<  const=0.05  OutDataTypeStr=boolean
  isDone : Outport  VectorParamsAs1DForOutWhenUnconnected=off
  wires:
  Velocity/1 -> Logical Operator/2
  Relative Distance/1 -> Logical Operator/1
  relative_distance/1 -> Relative Distance/1
  Logical Operator/1 -> isDone/1
  v_ego/1 -> Velocity/1

== system rlMADDPG4PFC2/ACCEL 3/Subsystem3 ==
  d_err : Inport
  v_ego : Inport  Port=2
  v_lead : Inport  Port=3
  Constant : Constant  Value=v_set
  Min : MinMax  Inputs=2
  Sum1 : Sum  Inputs=+-
  Switch : Switch  Criteria=u2 > Threshold  SaturateOnIntegerOverflow=off  InputSameDT=off
  v_err : Outport  VectorParamsAs1DForOutWhenUnconnected=off
  wires:
  Sum1/1 -> v_err/1
  v_ego/1 -> Sum1/2
  Switch/1 -> Sum1/1  "v_ref"
  d_err/1 -> Switch/2
  Constant/1 -> Min/2, Switch/3
  Min/1 -> Switch/1
  v_lead/1 -> Min/1

== system rlMADDPG4PFC2/Ego Vehicle and Environment1/Ego sensor ==
  Longitudinal velocity : Inport
  Lateral velocity : Inport  Port=2
  Yaw rate : Inport  Port=3
  Curvature : Inport  Port=4
  Initial relative yaw angle : Inport  Port=5
  Initial lateral deviation : Inport  Port=6
  Integrator : Integrator
  Integrator2 : Integrator
  Mux1 : Mux  Inputs=[1 1 1]
  Product : Product
  Subtract : Sum  Inputs=-+
  Sum : Sum
  Sum1 : Sum
  e1dot : Fcn  Expr=u(1)*u(3)+u(2)
  Lateral deviation : Outport  VectorParamsAs1DForOutWhenUnconnected=off
  Relative yaw angle : Outport  Port=2  VectorParamsAs1DForOutWhenUnconnected=off
  e1_dot : Outport  Port=3  VectorParamsAs1DForOutWhenUnconnected=off
  e2_dot : Outport  Port=4  VectorParamsAs1DForOutWhenUnconnected=off
  wires:
  Curvature/1 -> Product/2
  Sum1/1 -> Mux1/3, Relative yaw angle/1  "e2_2"
  Mux1/1 -> e1dot/1
  Initial lateral deviation/1 -> Sum/1
  e1dot/1 -> e1_dot/1, Integrator/1
  Integrator/1 -> Sum/2
  Longitudinal velocity/1 -> Product/1, Mux1/1
  Lateral velocity/1 -> Mux1/2
  Sum/1 -> Lateral deviation/1  "e1_2"
  Integrator2/1 -> Sum1/1
  Initial relative yaw angle/1 -> Sum1/2
  Product/1 -> Subtract/1
  Yaw rate/1 -> Subtract/2
  Subtract/1 -> e2_dot/1, Integrator2/1  "e2dot"

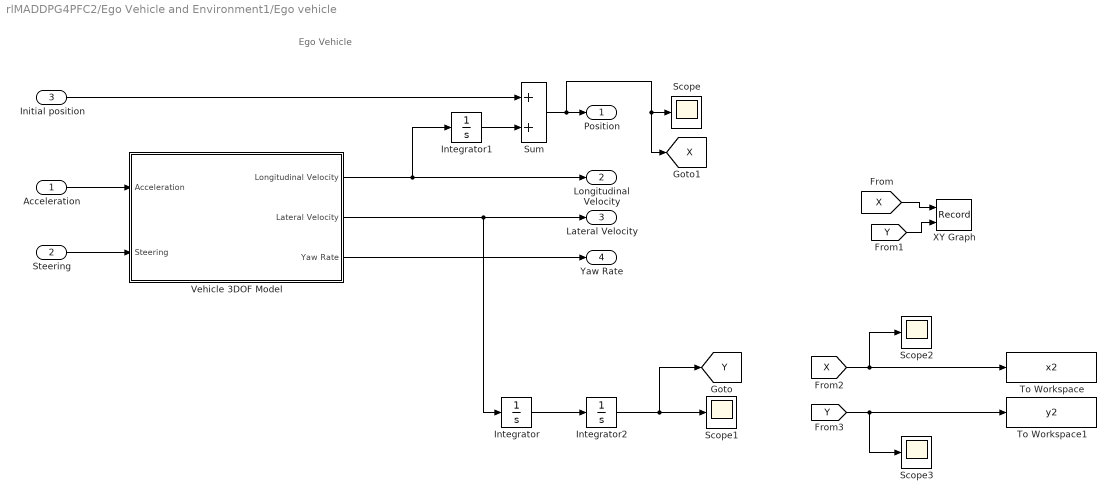
== system rlMADDPG4PFC2/Ego Vehicle and Environment1/Ego vehicle ==
  note: Ego Vehicle
  Acceleration : Inport
  Steering : Inport  Port=2
  Initial position : Inport  Port=3
  Integrator : Integrator
  Integrator1 : Integrator
  Integrator2 : Integrator
  Scope{,1..3} (4 alike) : Scope
  Sum : Sum
  To Workspace : ToWorkspace  VariableName=x2  SampleTime=-1
      settings: Save2DSignal=2-D array (concatenate along first dimension)
  To Workspace1 : ToWorkspace  VariableName=y2  SampleTime=-1
      settings: Save2DSignal=2-D array (concatenate along first dimension)
  Vehicle 3DOF Model : Subsystem
  XY Graph : Record  FileSettingsInternal="{\"entries\":[{\"content\":{\"excelSettings\":{\"content\":{},\"type\":\"Streamout.ExcelSettings\"}},\"type\":\"Streamout.FileSettingStorage\",\"uuid\":\"\"}],\"packageUris\":[\"http:\\/\\/schema.mathworks.com\\/mf0\\/streamout_blocks\\/R2020a\"],\"version\":\"1.0\"}"  Layout=[1 1]  SignalsInternal="{\"entries\":[{\"content\":{\"signals\":[{\"content\":{\"blockPath\":[],\"dimensions\":[1],\"domain\":\"\",\"lineColor\":\"#ff13a6\",\"lineWidth\":2,\"port\":1,\"sid\":[\"\"],\"signalID\":1,\"signalName\":\"From\"},\"type\":\"RecordBlkView.Signal\",\"uuid\":\"\"},{\"content\":{\"blockPath\":[],\"dimensions\":[1],\"domain\":\"\",\"lineColor\":\"#fe330a\",\"lineWidth\":2,\"plots\":[ 1 ],\"port\":2,\"sid\":[\"\"],\"signalID\":2,\"signalName\":\"From1\"},\"type\":\"RecordBlkView.Signal\",\"uuid\":\"\"}]},\"type\":\"RecordBlkView.InputSignals\",\"uuid\":\"\"}],\"packageUris\":[\"http:\\/\\/schema.mathworks.com\\/mf0\\/streamout_blocks\\/R2020a\"],\"version\":\"1.0\"}"  VisualizationBindings="{\"sparklinesplugin\":{\"info\":[{\"bindingParametersList\":[],\"subplotID\":1}]}}"  CompatibilityTag=XY
  Position : Outport  VectorParamsAs1DForOutWhenUnconnected=off
  Longitudinal Velocity : Outport  Port=2  VectorParamsAs1DForOutWhenUnconnected=off
  Lateral Velocity : Outport  Port=3  VectorParamsAs1DForOutWhenUnconnected=off
  Yaw Rate : Outport  Port=4  VectorParamsAs1DForOutWhenUnconnected=off
  tag scope: X=global, Y=global
  wires:
  Integrator1/1 -> Sum/2
  Initial position/1 -> Sum/1
  Acceleration/1 -> Vehicle 3DOF Model/1(Acceleration)
  Steering/1 -> Vehicle 3DOF Model/2(Steering)
  Vehicle 3DOF Model/3(Yaw Rate) -> Yaw Rate/1
  Vehicle 3DOF Model/1(Longitudinal Velocity) -> Longitudinal Velocity/1, Integrator1/1
  Sum/1 -> [X], Scope/1, Position/1
  Vehicle 3DOF Model/2(Lateral Velocity) -> Integrator/1, Lateral Velocity/1
  Integrator/1 -> Integrator2/1
  Integrator2/1 -> [Y], Scope1/1
  [X] -> XY Graph/1
  [Y] -> XY Graph/2
  [Y] -> To Workspace1/1, Scope3/1
  [X] -> Scope2/1, To Workspace/1

== system rlMADDPG4PFC2/Ego Vehicle and Environment1/curvature1 ==
  position : Inport
  Cos : Trigonometry  Operator=cos
  Derivative2 : Derivative
  Integrator : Integrator
  Integrator1 : Integrator
  Integrator2 : Integrator
  M-curve : MATLAB Function  TreatAsAtomicUnit=on
  Multiport Switch : MultiPortSwitch  SaturateOnIntegerOverflow=off  InputSameDT=off
  N-curve : MATLAB Function  TreatAsAtomicUnit=on
  Product : Product
  Product1 : Product
  Product2 : Product
  S-curve : MATLAB Function  TreatAsAtomicUnit=on
  Scope : Scope
  Sin : Trigonometry
  XY Graph : Record  FileSettingsInternal="{\"entries\":[{\"content\":{\"excelSettings\":{\"content\":{},\"type\":\"Streamout.ExcelSettings\"}},\"type\":\"Streamout.FileSettingStorage\",\"uuid\":\"\"}],\"packageUris\":[\"http:\\/\\/schema.mathworks.com\\/mf0\\/streamout_blocks\\/R2020a\"],\"version\":\"1.0\"}"  Layout=[1 1]  SignalsInternal="{\"entries\":[{\"content\":{\"signals\":[{\"content\":{\"blockPath\":[],\"dimensions\":[1],\"domain\":\"\",\"lineColor\":\"#d95319\",\"lineWidth\":2,\"port\":1,\"sid\":[\"\"],\"signalID\":1,\"signalName\":\"Integrator1\"},\"type\":\"RecordBlkView.Signal\",\"uuid\":\"\"},{\"content\":{\"blockPath\":[],\"dimensions\":[1],\"domain\":\"\",\"lineColor\":\"#edb120\",\"lineWidth\":2,\"port\":2,\"sid\":[\"\"],\"signalID\":2,\"signalName\":\"Integrator2\"},\"type\":\"RecordBlkView.Signal\",\"uuid\":\"\"}]},\"type\":\"RecordBlkView.InputSignals\",\"uuid\":\"\"}],\"packageUris\":[\"http:\\/\\/schema.mathworks.com\\/mf0\\/streamout_blocks\\/R2020a\"],\"version\":\"1.0\"}"  VisualizationBindings="{\"xyplotplugin\":{\"info\":[{\"series\":[],\"subplotID\":1}]}}"  CompatibilityTag=XY
  work condition : Constant  Value=target
  curvature : Outport
  wires:
  Integrator1/1 -> XY Graph/1
  Integrator2/1 -> XY Graph/2
  Integrator/1 -> Cos/1, Sin/1
  Derivative2/1 -> Product1/2, Product2/1, Product/2
  Product/1 -> Integrator/1
  Product2/1 -> Integrator2/1
  Sin/1 -> Product2/2
  Product1/1 -> Integrator1/1
  Cos/1 -> Product1/1
  position/1 -> S-curve/1(s), Derivative2/1, M-curve/1(s), N-curve/1(s)
  Multiport Switch/1 -> Product/1, curvature/1, Scope/1
  S-curve/1(rho) -> Multiport Switch/2
  N-curve/1(rho) -> Multiport Switch/3
  work condition/1 -> Multiport Switch/1
  M-curve/1(rho) -> Multiport Switch/4

== system rlMADDPG4PFC2/Ego Vehicle and Environment3/Ego sensor ==
  Longitudinal velocity : Inport
  Lateral velocity : Inport  Port=2
  Yaw rate : Inport  Port=3
  Curvature : Inport  Port=4
  Initial relative yaw angle : Inport  Port=5
  Initial lateral deviation : Inport  Port=6
  Integrator : Integrator
  Integrator2 : Integrator
  Mux1 : Mux  Inputs=[1 1 1]
  Product : Product
  Subtract : Sum  Inputs=-+
  Sum : Sum
  Sum1 : Sum
  e1dot : Fcn  Expr=u(1)*u(3)+u(2)
  Lateral deviation : Outport  VectorParamsAs1DForOutWhenUnconnected=off
  Relative yaw angle : Outport  Port=2  VectorParamsAs1DForOutWhenUnconnected=off
  e1_dot : Outport  Port=3  VectorParamsAs1DForOutWhenUnconnected=off
  e2_dot : Outport  Port=4  VectorParamsAs1DForOutWhenUnconnected=off
  wires:
  Curvature/1 -> Product/2
  Sum1/1 -> Mux1/3, Relative yaw angle/1  "e2_1"
  Mux1/1 -> e1dot/1
  Initial lateral deviation/1 -> Sum/1
  e1dot/1 -> e1_dot/1, Integrator/1
  Integrator/1 -> Sum/2
  Longitudinal velocity/1 -> Product/1, Mux1/1
  Lateral velocity/1 -> Mux1/2
  Sum/1 -> Lateral deviation/1  "e1_1"
  Integrator2/1 -> Sum1/1
  Initial relative yaw angle/1 -> Sum1/2
  Product/1 -> Subtract/1
  Yaw rate/1 -> Subtract/2
  Subtract/1 -> e2_dot/1, Integrator2/1  "e2dot"

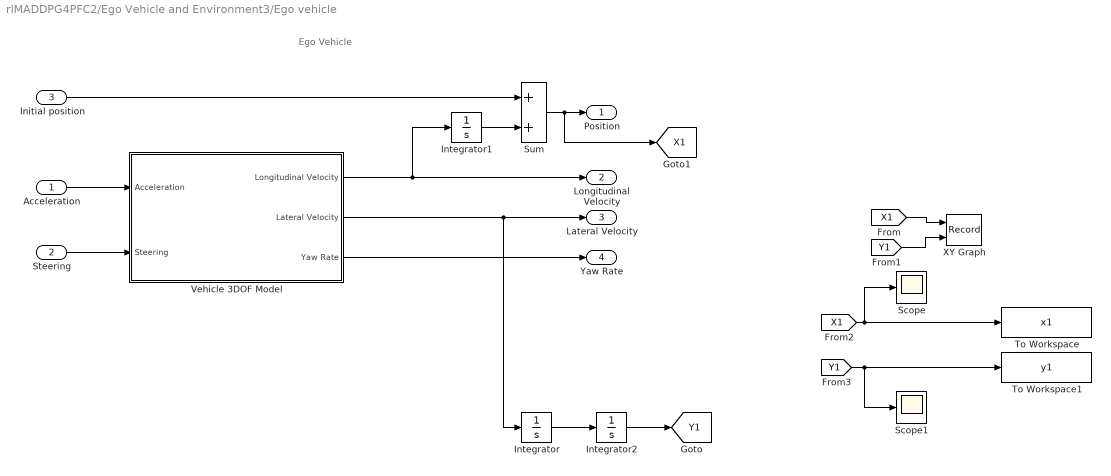
== system rlMADDPG4PFC2/Ego Vehicle and Environment3/Ego vehicle ==
  note: Ego Vehicle
  Acceleration : Inport
  Steering : Inport  Port=2
  Initial position : Inport  Port=3
  Integrator : Integrator
  Integrator1 : Integrator
  Integrator2 : Integrator
  Scope : Scope
  Scope1 : Scope
  Sum : Sum
  To Workspace : ToWorkspace  VariableName=x1  SampleTime=-1
      settings: Save2DSignal=2-D array (concatenate along first dimension)
  To Workspace1 : ToWorkspace  VariableName=y1  SampleTime=-1
      settings: Save2DSignal=2-D array (concatenate along first dimension)
  Vehicle 3DOF Model : Subsystem
  XY Graph : Record  FileSettingsInternal="{\"entries\":[{\"content\":{\"excelSettings\":{\"content\":{},\"type\":\"Streamout.ExcelSettings\"}},\"type\":\"Streamout.FileSettingStorage\",\"uuid\":\"\"}],\"packageUris\":[\"http:\\/\\/schema.mathworks.com\\/mf0\\/streamout_blocks\\/R2020a\"],\"version\":\"1.0\"}"  Layout=[1 1]  SignalsInternal="{\"entries\":[{\"content\":{\"signals\":[{\"content\":{\"blockPath\":[],\"dimensions\":[1],\"domain\":\"\",\"lineColor\":\"#d95319\",\"lineWidth\":2,\"port\":1,\"sid\":[\"\"],\"signalID\":1,\"signalName\":\"From\"},\"type\":\"RecordBlkView.Signal\",\"uuid\":\"\"},{\"content\":{\"blockPath\":[],\"dimensions\":[1],\"domain\":\"\",\"lineColor\":\"#edb120\",\"lineWidth\":2,\"plots\":[ 1 ],\"port\":2,\"sid\":[\"\"],\"signalID\":2,\"signalName\":\"From1\"},\"type\":\"RecordBlkView.Signal\",\"uuid\":\"\"}]},\"type\":\"RecordBlkView.InputSignals\",\"uuid\":\"\"}],\"packageUris\":[\"http:\\/\\/schema.mathworks.com\\/mf0\\/streamout_blocks\\/R2020a\"],\"version\":\"1.0\"}"  VisualizationBindings="{\"sparklinesplugin\":{\"info\":[{\"bindingParametersList\":[],\"subplotID\":1}]}}"  CompatibilityTag=XY
  Position : Outport  VectorParamsAs1DForOutWhenUnconnected=off
  Longitudinal Velocity : Outport  Port=2  VectorParamsAs1DForOutWhenUnconnected=off
  Lateral Velocity : Outport  Port=3  VectorParamsAs1DForOutWhenUnconnected=off
  Yaw Rate : Outport  Port=4  VectorParamsAs1DForOutWhenUnconnected=off
  tag scope: X1=global, Y1=global
  wires:
  Integrator1/1 -> Sum/2
  Initial position/1 -> Sum/1
  Acceleration/1 -> Vehicle 3DOF Model/1(Acceleration)
  Steering/1 -> Vehicle 3DOF Model/2(Steering)
  Vehicle 3DOF Model/3(Yaw Rate) -> Yaw Rate/1
  Vehicle 3DOF Model/1(Longitudinal Velocity) -> Longitudinal Velocity/1, Integrator1/1
  Vehicle 3DOF Model/2(Lateral Velocity) -> Integrator/1, Lateral Velocity/1
  Sum/1 -> [X1], Position/1
  Integrator2/1 -> [Y1]
  Integrator/1 -> Integrator2/1
  [X1] -> XY Graph/1
  [Y1] -> XY Graph/2
  [X1] -> Scope/1, To Workspace/1
  [Y1] -> To Workspace1/1, Scope1/1

== system rlMADDPG4PFC2/Ego Vehicle and Environment3/Lead vehicle1 ==
  Initial position : Inport
  Initial velocity : Inport  Port=2
  Constant : Constant  Value=target
  Integrator : Integrator
  Integrator1 : Integrator
  Multiport Switch1 : MultiPortSwitch  SaturateOnIntegerOverflow=off  InputSameDT=off
  Sine1 : Sin  Amplitude=0.05  Frequency=2*pi/60  SampleTime=Ts
  Sum : Sum
  Sum1 : Sum
  Transfer Fcn : TransferFcn  Denominator=[0.6 1]
  a_LV : Scope
  ramp1 : Subsystem
  step1 : Subsystem
  Position : Outport  VectorParamsAs1DForOutWhenUnconnected=off
  Longitudinal velocity : Outport  Port=2  VectorParamsAs1DForOutWhenUnconnected=off
  a_lead : Outport  Port=3  VectorParamsAs1DForOutWhenUnconnected=off
  wires:
  Transfer Fcn/1 -> Sum1/1
  Initial velocity/1 -> Sum1/2
  Sum/1 -> Position/1
  Integrator/1 -> Transfer Fcn/1
  Sum1/1 -> Integrator1/1, Longitudinal velocity/1
  Initial position/1 -> Sum/1
  Integrator1/1 -> Sum/2
  Sine1/1 -> Multiport Switch1/3  "a_LV"
  ramp1/1(Out1) -> Multiport Switch1/2
  step1/1(a_LV) -> Multiport Switch1/4
  Multiport Switch1/1 -> a_lead/1, a_LV/1, Integrator/1  "a_LV"
  Constant/1 -> Multiport Switch1/1

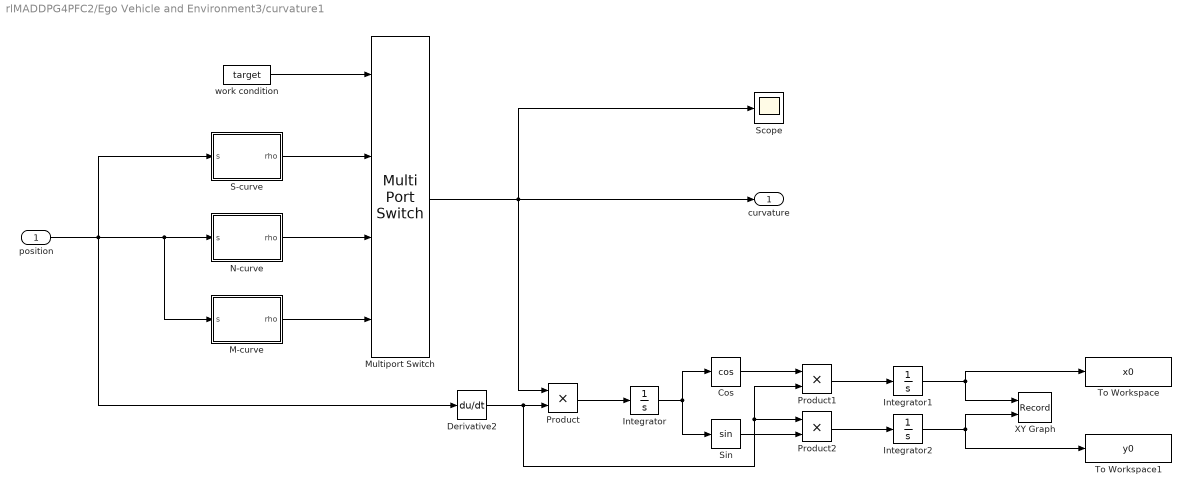
== system rlMADDPG4PFC2/Ego Vehicle and Environment3/curvature1 ==
  position : Inport
  Cos : Trigonometry  Operator=cos
  Derivative2 : Derivative
  Integrator : Integrator
  Integrator1 : Integrator
  Integrator2 : Integrator
  M-curve : MATLAB Function  TreatAsAtomicUnit=on
  Multiport Switch : MultiPortSwitch  SaturateOnIntegerOverflow=off  InputSameDT=off
  N-curve : MATLAB Function  TreatAsAtomicUnit=on
  Product : Product
  Product1 : Product
  Product2 : Product
  S-curve : MATLAB Function  TreatAsAtomicUnit=on
  Scope : Scope
  Sin : Trigonometry
  To Workspace : ToWorkspace  VariableName=x0  SampleTime=-1
      settings: Save2DSignal=2-D array (concatenate along first dimension)
  To Workspace1 : ToWorkspace  VariableName=y0  SampleTime=-1
      settings: Save2DSignal=2-D array (concatenate along first dimension)
  XY Graph : Record  FileSettingsInternal="{\"entries\":[{\"content\":{\"excelSettings\":{\"content\":{},\"type\":\"Streamout.ExcelSettings\"}},\"type\":\"Streamout.FileSettingStorage\",\"uuid\":\"\"}],\"packageUris\":[\"http:\\/\\/schema.mathworks.com\\/mf0\\/streamout_blocks\\/R2020a\"],\"version\":\"1.0\"}"  Layout=[1 1]  SignalsInternal="{\"entries\":[{\"content\":{\"signals\":[{\"content\":{\"blockPath\":[],\"dimensions\":[1],\"domain\":\"\",\"lineColor\":\"#139fff\",\"lineWidth\":2,\"port\":1,\"sid\":[\"\"],\"signalID\":1,\"signalName\":\"Integrator1\"},\"type\":\"RecordBlkView.Signal\",\"uuid\":\"\"},{\"content\":{\"blockPath\":[],\"dimensions\":[1],\"domain\":\"\",\"lineColor\":\"#ff6929\",\"lineWidth\":2,\"port\":2,\"sid\":[\"\"],\"signalID\":2,\"signalName\":\"Integrator2\"},\"type\":\"RecordBlkView.Signal\",\"uuid\":\"\"}]},\"type\":\"RecordBlkView.InputSignals\",\"uuid\":\"\"}],\"packageUris\":[\"http:\\/\\/schema.mathworks.com\\/mf0\\/streamout_blocks\\/R2020a\"],\"version\":\"1.0\"}"  VisualizationBindings="{\"xyplotplugin\":{\"info\":[{\"series\":[],\"subplotID\":1}]}}"  CompatibilityTag=XY
  work condition : Constant  Value=target
  curvature : Outport
  wires:
  Integrator2/1 -> To Workspace1/1, XY Graph/2
  Integrator/1 -> Cos/1, Sin/1
  Derivative2/1 -> Product1/2, Product2/1, Product/2
  Product/1 -> Integrator/1
  Product2/1 -> Integrator2/1
  Sin/1 -> Product2/2
  Product1/1 -> Integrator1/1
  Cos/1 -> Product1/1
  position/1 -> S-curve/1(s), Derivative2/1, M-curve/1(s), N-curve/1(s)
  Multiport Switch/1 -> Product/1, curvature/1, Scope/1
  S-curve/1(rho) -> Multiport Switch/2
  N-curve/1(rho) -> Multiport Switch/3
  work condition/1 -> Multiport Switch/1
  M-curve/1(rho) -> Multiport Switch/4
  Integrator1/1 -> To Workspace/1, XY Graph/1

== system rlMADDPG4PFC2/STEER2/Subsystem ==
  steer : Inport
  e1 : Inport  Port=2
  Compare To Constant1 : simulink/Logic and Bit Operations/Compare To Constant  relop=<  const=0.01  OutDataTypeStr=boolean
  Gain : Gain  Gain=0.1
  Gain2 : Gain  Gain=0.5
  Gain5 : Gain  Gain=2
  Square : Math  Operator=square  SignedPower=on
  Square2 : Math  Operator=square  SignedPower=on
  Sum1 : Sum  Inputs=-++
  Unit Delay : UnitDelay  SampleTime=-1  HasFrameUpgradeWarning=on
  Cost : Outport  VectorParamsAs1DForOutWhenUnconnected=off
  wires:
  e1/1 -> Square/1
  Sum1/1 -> Cost/1
  Gain/1 -> Sum1/2
  steer/1 -> Unit Delay/1
  Square2/1 -> Gain2/1
  Gain2/1 -> Sum1/3
  Unit Delay/1 -> Square2/1
  Compare To Constant1/1 -> Gain5/1
  Square/1 -> Compare To Constant1/1, Gain/1
  Gain5/1 -> Sum1/1

== system rlMADDPG4PFC2/STEER2/Subsystem1 ==
  e1 : Inport
  e2 : Inport  Port=2
  e1dot : Inport  Port=3
  e2dot : Inport  Port=4
  steer1 : Inport  Port=5
  lat1 : Inport  Port=6
  yaw1 : Inport  Port=7
  Discrete-Time Integrator : DiscreteIntegrator  SampleTime=-1  ICPrevOutput=DiscIntNeverNeededParam  ICPrevScaledInput=DiscIntNeverNeededParam
  Discrete-Time Integrator1 : DiscreteIntegrator  SampleTime=-1  ICPrevOutput=DiscIntNeverNeededParam  ICPrevScaledInput=DiscIntNeverNeededParam
  Mux : Mux  Inputs=9
  obs : Outport  VectorParamsAs1DForOutWhenUnconnected=off
  wires:
  e1/1 -> Mux/2, Discrete-Time Integrator1/1
  Mux/1 -> obs/1
  Discrete-Time Integrator1/1 -> Mux/1  "integral_error"
  e2/1 -> Mux/4, Discrete-Time Integrator/1
  Discrete-Time Integrator/1 -> Mux/3  "integral_error"
  e1dot/1 -> Mux/5
  e2dot/1 -> Mux/6
  steer1/1 -> Mux/7
  lat1/1 -> Mux/8
  yaw1/1 -> Mux/9
